simulink model "px4demo_gps"  (R2016b)
settings: Solver=ode3  StartTime=0.0  StopTime=inf  FixedStep=1/250  RelTol=1e-3
PostLoadFcn:
  | Ts = 1/250;
undefined symbols (not defined in the file or in its folder): RGBLED_COLOR_ENUM, RGBLED_MODE_ENUM
libraries: pixhawk_slib_sensors_actuators x2, pixhawk_slib_ADC_serial x1
settings Model: Creator=skuznick  LastModifiedBy=E6320
settings DataIOCC: LimitDataPoints=on  SaveFormat=Array
settings OptimizationCC: DefaultParameterBehavior=Inlined  LifeSpan=1  MaxStackSize=64
settings DebuggingCC: SolverPrmCheckMsg=warning  AllowSymbolicDim=off  SFUnexpectedBacktrackingDiag=warning  SFNoUnconditionalDefaultTransitionDiag=warning  SFExecutionAtInitializationDiag=none
settings HardwareCC: ProdBitPerPointer=32  ProdBitPerSizeT=32  ProdBitPerPtrDiffT=32  ProdLargestAtomicInteger=Long  ProdLargestAtomicFloat=Double  ProdWordSize=32  ProdHWDeviceType=ARM Compatible->ARM Cortex
settings ModelReferenceCC: PropagateSignalLabelsOutOfModel=off
settings RTWCC: SystemTargetFile=ert.tlc  HardwareBoard=Pixhawk PX4  TemplateMakefile=ert_default_tmf  Description=Embedded Coder  GenerateReport=on  Toolchain=Pixhawk Toolchain  IncludeHyperlinkInReport=on  LaunchReport=on  GenerateTraceReport=on  GenerateCodeMetricsReport=on
settings CodeAppCC: IgnoreCustomStorageClasses=off
settings ERTTargetCC: ERTCustomFileTemplate=PX4_codertarget_file_process.tlc  ConvertIfToSwitch=off  SuppressUnreachableDefaultCases=off
settings ConfigComp: CovMetricSettings=dw  CovHtmlReporting=on  CovSaveCumulativeToWorkspaceVar=on  CovSaveSingleToWorkspaceVar=on  CovExternalEMLEnable=off  CovSFcnEnable=off

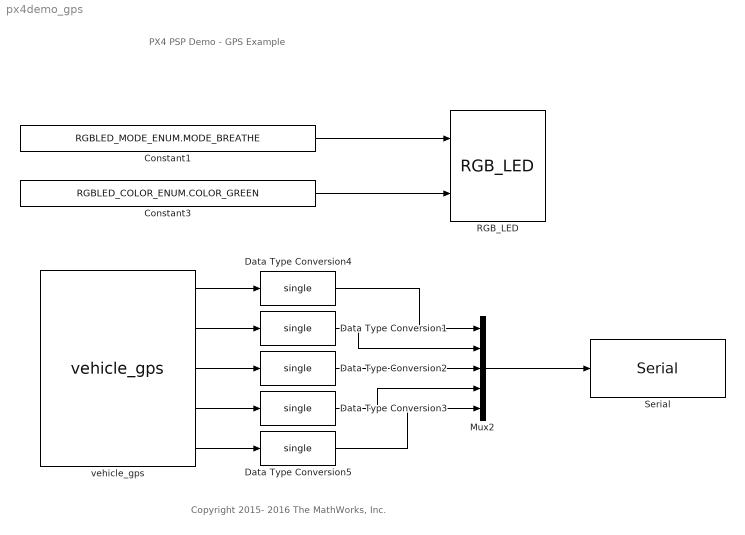
== system px4demo_gps ==
  note: Copyright 2015- 2016 The MathWorks, Inc.
  note: PX4 PSP Demo - GPS Example
  Constant1 : Constant  Value=RGBLED_MODE_ENUM.MODE_BREATHE  OutDataTypeStr=Enum: RGBLED_MODE_ENUM  SampleTime=Ts
  Constant3 : Constant  Value=RGBLED_COLOR_ENUM.COLOR_GREEN  OutDataTypeStr=Enum: RGBLED_COLOR_ENUM  SampleTime=Ts
  Data Type Conversion{1..5} (5 alike) : DataTypeConversion  OutDataTypeStr=single
  Mux2 : Mux  Inputs=5
  RGB_LED : pixhawk_slib_sensors_actuators/RGB_LED
  Serial : pixhawk_slib_ADC_serial/Serial  DeviceName=/dev/ttyS1  ReadOrWrite=Writing  BaudRateStr=57600  block=on  WriteStatus=on  Terminator=off  Header=on  NumBytesRead=4  TerminatorChar=\n  HeaderData=[ uint8( hex2dec( 'DE' ) ), uint8( hex2dec( 'AD' ) ), uint8( hex2dec( 'C0' ) ), uint8( hex2dec( 'DE' ) ) ]  SimulateUsing=Code generation
  vehicle_gps : pixhawk_slib_sensors_actuators/vehicle_gps  sampletime=Ts  show_ts_pos=off  show_alt=on  show_ts_gps=off  show_vel=off  show_fixtype=on  show_numsat=on
  wires:
  Constant1/1 -> RGB_LED/1
  Constant3/1 -> RGB_LED/2
  Mux2/1 -> Serial/1
  vehicle_gps/1 -> Data Type Conversion4/1
  vehicle_gps/2 -> Data Type Conversion1/1
  vehicle_gps/3 -> Data Type Conversion2/1
  vehicle_gps/5 -> Data Type Conversion5/1
  Data Type Conversion4/1 -> Mux2/1
  Data Type Conversion1/1 -> Mux2/2
  Data Type Conversion2/1 -> Mux2/3
  Data Type Conversion3/1 -> Mux2/4
  vehicle_gps/4 -> Data Type Conversion3/1
  Data Type Conversion5/1 -> Mux2/5
